simulink model "GCU_Model_genCode"  (R2018a)
settings: Solver=FixedStepDiscrete  StartTime=0.0  StopTime=20  FixedStep=0.0001  RelTol=1e-3  EnableMultiTasking=on
undefined symbols (not defined in the file): ConversionGainVector, ConversionOffsetVector, VoltageGainVector, VoltageOffsetVector
libraries: canLib x5, simulink x5, uartLib x2, utilityLib x1, clutchMotorLib x1, efiLib x1, engineControlLib x1, cstblocks x1, gearMotorLib x1
(part 2 of 3)

== system GCU_Model_genCode/EEPROM/Evaluate_Request/Read ==
  page : Inport
  cell : Inport  Port=2
  dataSize : Inport  Port=3
  Action Port : ActionPort  ActionType=elseif
  Eeprom_read : S-Function  FunctionName=Eeprom_read  SFunctionDeploymentMode=off  EnableBusSupport=off
  readResult : Outport
  data : Outport  Port=2
  wires:
  Eeprom_read/1 -> readResult/1
  Eeprom_read/2 -> data/1
  page/1 -> Eeprom_read/1
  cell/1 -> Eeprom_read/2
  dataSize/1 -> Eeprom_read/3

== system GCU_Model_genCode/EEPROM/Evaluate_Request/Write ==
  page : Inport
  cell : Inport  Port=2
  dataSize : Inport  Port=3
  data : Inport  Port=4
  Action Port : ActionPort  ActionType=then
  Eeprom_write : S-Function  FunctionName=Eeprom_write  SFunctionDeploymentMode=off  EnableBusSupport=off
  writeResult : Outport
  wpState : Outport  Port=2
  wires:
  cell/1 -> Eeprom_write/2
  page/1 -> Eeprom_write/1
  dataSize/1 -> Eeprom_write/3
  data/1 -> Eeprom_write/4
  Eeprom_write/2 -> wpState/1
  Eeprom_write/1 -> writeResult/1

== system GCU_Model_genCode/GCU_CAN_Read/MessageEvaluation1/setMap/If Action Subsystem ==
  In1 : Inport
  Action Port : ActionPort  ActionType=then
  Out1 : Outport
  wires:
  In1/1 -> Out1/1

== system GCU_Model_genCode/GCU_CAN_Read/MessageEvaluation1/setMap/If Action Subsystem1 ==
  In1 : Inport
  Action Port : ActionPort  ActionType=else
  Out1 : Outport
  wires:
  In1/1 -> Out1/1

== system GCU_Model_genCode/GCU_timer/Anti_Stall_System/antiStallLogic/AntiStallActivate ==
  Inport : Inport
  f : TriggerPort  TriggerType=function-call  VariantControl=(inherit)
      settings: CopyFcn=Stateflow.SLINSF.SimulinkMan.removeBlockPreDeleteFcn  PreDeleteFcn=Stateflow.SLINSF.SimulinkMan.unsafePredeleteFcn
  ClutchMotor SetPosition : S-Function  FunctionName=ClutchMotor_setPosition  SFunctionDeploymentMode=off  EnableBusSupport=off
  wires:
  Inport/1 -> ClutchMotor SetPosition/1

== stateflow chart GCU_Model_genCode/GCU_timer/GCULogic ==
  settings: updateMethod=DISCRETE  sampleTime=0.001
  state MODES [parallel]
    settings: executionOrder=1
    state MANUAL_MODES
      entry:
      lastModeCom[0] = modeCom[0];
      lastModeCom[1] = modeCom[1];
      entry, during:
      checkShift();
      checkClutch();
      state ENDURANCE
      state SKIDPAD
      (default) -> ENDURANCE
    state INIT
      entry:
      send(BuzzerOn);
      during:
      buzzerCounter++;
    note: azzerare nel modo giusto i feedback e i comandi
    note: POSSIAMO FARLO UGUALE PER ACCELERATION E AUTOX?
    state checkClutch [function]
      (default) -> (junction 649)
      (junction 649) -> (junction 648) [order 1] : [clutchTarget ~= clutchCurrVal && antiStallFb == ANTISTALL_OFF]
      (junction 649) -> (junction 683) [order 2]
      (junction 648) -> (junction 682)
      (junction 682) -> (junction 687) [order 1] : [(~in(GEARSHIFT.DOWNSHIFTING) && ~in(NEUTRAL_STATE.SET_NEUTRAL)) || in(NEUTRAL_STATE.UNSET_NEUTRAL)]
      (junction 682) -> (junction 689) [order 2]
      (junction 687) -> (junction 691) : {Clutch_setValue(clutchTarget);}
    note: In caso di problema si riporta in endurance
    state checkShift [function]
      (default) -> (junction 635)
      (junction 635) -> (junction 637) [order 1] : [shiftCom[0] ~= lastShiftCom]
      (junction 635) -> (junction 641) [order 2]
      (junction 637) -> (junction 448) : {lastShiftCom = shiftCom[0];}
      (junction 448) -> (junction 450) [order 1] : [ shiftCom[1] == GEAR_COMMAND_UP]
      (junction 448) -> (junction 454) [order 2]
      (junction 450) -> (junction 452) : {send(GearshiftUp, NEUTRAL_STATE);
          |  send(GearshiftUp, GEARSHIFT);}
      (junction 454) -> (junction 456) [order 1] : [shiftCom[1] == GEAR_COMMAND_DOWN]
      (junction 454) -> (junction 460) [order 2]
      (junction 456) -> (junction 458) : {send(GearshiftDown, NEUTRAL_STATE);
          |  send(GearshiftDown, GEARSHIFT);}
      (junction 460) -> (junction 462) [order 1] : [shiftCom[1] == GEAR_COMMAND_NEUTRAL_UP]
      (junction 460) -> (junction 466) [order 2]
      (junction 462) -> (junction 464) : {send(GearshiftSetNeutral, NEUTRAL_STATE);
          |  send(GearshiftUp, GEARSHIFT);}
      (junction 466) -> (junction 469) [order 1] : [shiftCom[1] == GEAR_COMMAND_NEUTRAL_DOWN]
      (junction 466) -> (junction 473) [order 2]
      (junction 469) -> (junction 471) : {send(GearshiftSetNeutral, NEUTRAL_STATE);
          |  send(GearshiftDown, GEARSHIFT); }
    state ACCELERATION
      entry:
      lastAacCom = aacCom[0];
      lastModeCom[0] = modeCom[0];
      lastModeCom[1] = modeCom[1];
      note: ClutchSet si annulla se provo a tirarla in ready?
      state ACC
        note: Ricorda load dei default parameters
        note: Forse serve stato OFF, forse no
        note: ATTENZIONE: mancano delle istruzioni in alcuni stati
        note: E' giusto che clutch venga settata due volte?
        note: Riguarda funzionamento counter
        state ACTIVE
          note: Quindi continuo a settare Clutch?
          state START
            entry:
            stateFb = ACC_READY;
            aacCounter = AAC_WORK_RATE_ms
            send(Efi_setRPMLimiter);
            Clutch_setValue(uint8(100));
            during:
            aacCounter = aacCounter - 1;
          state READY
            entry:
            stateFb = ACC_READY;
            aacCounter = AAC_WORK_RATE_ms
            Clutch_setValue(uint8(100));
            during:
            aacCounter = aacCounter - 1;
            en, du:
            checkShift();
          note: SET blip è sbagliato
          state START_RELEASE
            entry:
            stateFb = ACC_GO;
            aac_clutchValue = double(getAacParam(acc_params.RAMP_START));
            Clutch_setValue(uint8(aac_clutchValue));
            aac_dtRelease = getAacParam(acc_params.RAMP_TIME) / int32(AAC_WORK_RATE_ms);
            aac_clutchStep = double((getAacParam(acc_params.RAMP_START) - getAacParam(acc_params.RAMP_END)) * int32(AAC_WORK_RATE_ms)) / double(getAacParam(acc_params.RAMP_TIME));
            aacCounter = AAC_WORK_RATE_ms;
            during:
            aacCounter = aacCounter - 1;
          state RUNNING
            entry:
            aacCounter = AAC_WORK_RATE_ms
            lastShift =  currentGear;
            entry, during:
            aacCheckShift();
          note: Continuo a controllare ogni 25ms?
          state aacCheckShift [function]
            (default) -> (junction 716)
            (junction 716) -> (junction 717) [order 1] : [lastShift == currentGear]
            (junction 716) -> (junction 720) [order 2]
            (junction 717) -> (junction 593)
            (junction 593) -> (junction 604) [order 1] : [acc_externValues[int32(acc_values.RPM)] >= acc_parameters[ uint8(acc_params.RPM_LIMIT_1_2) + currentGear -1]]
            (junction 593) -> (junction 606) [order 2]
            (junction 604) -> (junction 608)
            (junction 608) -> (junction 610) [order 1] : [acc_externValues[int32(acc_values.WHEEL_SPEED)] >= acc_parameters[ uint8(acc_params.SPEED_LIMIT_1_2) + currentGear-1]]
            (junction 608) -> (junction 612) [order 2]
            (junction 610) -> (junction 614) : {send(GearshiftUp, GEARSHIFT); lastShift = lastShift + 1;}
          state RELEASING
            entry:
            aac_clutchValue = aac_clutchValue - aac_clutchStep;
            Clutch_setValue(uint8(aac_clutchValue));
            aac_dtRelease = aac_dtRelease - 1;
            aacCounter = AAC_WORK_RATE_ms;
            during:
            aacCounter = aacCounter - 1;
          note: Teniamo questa cosa di eseguire ogni 25ms? O calcoliamo direttamente
              | il Ttot?
          (default) -> MODES.ACCELERATION.ACC.ACTIVE.START
          (junction 558) -> MODES.ACCELERATION.ACC.ACTIVE.READY [order 2]
          MODES.ACCELERATION.ACC.ACTIVE.START -> MODES.ACCELERATION.ACC.ACTIVE.READY : [aacCounter <= 1]
          MODES.ACCELERATION.ACC.ACTIVE.READY -> (junction 558) : [aacCounter <= 1]
          (junction 558) -> MODES.ACCELERATION.ACC.ACTIVE.START_RELEASE [order 1] : [aacCom[0] ~= lastAacCom && aacCom[1] == ACC_GO && acc_externValues[int32(acc_values.TPS)] >= getAacParam(acc_params.TPS_START_LIMIT) ]{lastAacCom = aacCom[0];}
          MODES.ACCELERATION.ACC.ACTIVE.START_RELEASE -> MODES.ACCELERATION.ACC.ACTIVE.RELEASING : [aacCounter <= 1]
          (junction 572) -> MODES.ACCELERATION.ACC.ACTIVE.RUNNING [order 1] : [aac_dtRelease <= 0 || clutchCurrVal <= getAacParam(acc_params.RAMP_END)]
              | {Clutch_setValue(uint8(0)); send(Efi_unsetRPMLimiter);}
          (junction 572) -> MODES.ACCELERATION.ACC.ACTIVE.RELEASING [order 2]
          MODES.ACCELERATION.ACC.ACTIVE.RELEASING -> (junction 572) : [aacCounter <=1]
        note: Quando devo fare clutch release?Forse risolto in CAN
        state STOPPING
          entry:
          send(Efi_unsetRPMLimiter);
          Clutch_setValue(uint8(0));
          //sendUpdatesSW(ACC_CODE, uint16(0));
        note: da verificare la marcia di uscita
        note: !!!!Gli array di MATLAB sono 1-based
        state param = getAacParam(index) [function]
          (default) -> (junction 566)
          (junction 566) -> (junction 570) : {param = acc_parameters[int32(index)]}
        MODES.ACCELERATION.ACC.ACTIVE -> MODES.ACCELERATION.ACC.STOPPING : [aacCom[0] ~= lastAacCom && aacCom[1] == ACC_OFF]
            | {lastAacCom = aacCom[0]}
        MODES.ACCELERATION.ACC.ACTIVE.RUNNING -> MODES.ACCELERATION.ACC.STOPPING : [currentGear >= 5 && currentGear != 8]
      state DEFAULT
        entry, during:
        stateFb = ACC_OFF;
        checkShift();
        checkClutch();
      note: prima di entrare svuotare il buffer
      (default) -> MODES.ACCELERATION.DEFAULT
      MODES.ACCELERATION.DEFAULT -> MODES.ACCELERATION.ACC.ACTIVE : [aacCom[0] ~= lastAacCom && aacCom[1] == ACC_READY]
          | {lastAacCom = aacCom[0]}
      MODES.ACCELERATION.ACC.STOPPING -> MODES.ACCELERATION.DEFAULT
    note: il controllo se fare stopAcc in caso di comando di cambio meglio farlo dentro aac e non in CAN evaluation
    state AUTOCROSS
      entry:
      lastAutoXCom = autoXCom[0];
      lastModeCom[0] = modeCom[0];
      lastModeCom[1] = modeCom[1];
      state LAUNCH
        note: Ricorda load dei default parameters
        note: Forse serve stato OFF, forse no
        state ACTIVE
          note: TOGLIAMO STA COSA DEL WORK RATE?
          state START
            entry:
            stateFb = AUTOX_READY;
            autoXCounter = AUTOX_WORK_RATE_ms
            send(Efi_setRPMLimiter);
            Clutch_setValue(uint8(100));
            during:
            autoXCounter = autoXCounter - 1;
          state READY
            entry:
            stateFb = AUTOX_READY;
            autoXCounter = AUTOX_WORK_RATE_ms
            Clutch_setValue(uint8(100));
            during:
            autoXCounter = autoXCounter - 1;
            en, du:
            checkShift();
          state START_RELEASE
            entry:
            stateFb = AUTOX_GO;
            autoX_clutchValue = double(getAutoXParam(AUTOX_RAMP_START));
            Clutch_setValue(uint8(autoX_clutchValue));
            autoX_dtRelease = getAutoXParam(AUTOX_RAMP_TIME) / int32(AUTOX_WORK_RATE_ms);
            autoX_clutchStep = double((getAutoXParam(AUTOX_RAMP_START) - getAutoXParam(AUTOX_RAMP_END)) * int32(AUTOX_WORK_RATE_ms)) / double(getAutoXParam(AUTOX_RAMP_TIME));
            autoXCounter = AUTOX_WORK_RATE_ms;
            during:
            autoXCounter = autoXCounter - 1;
          state RUNNING
            entry:
            autoXCounter = AUTOX_WORK_RATE_ms
            lastShift =  currentGear;
            entry, during:
            autoXCheckShift();
          state autoXCheckShift [function]
            (default) -> (junction 1005)
            (junction 1005) -> (junction 1006) [order 1] : [lastShift == currentGear]
            (junction 1005) -> (junction 1007) [order 2]
            (junction 1006) -> (junction 1008)
            (junction 1008) -> (junction 1009) [order 1] : [acc_externValues[int32(acc_values.RPM)] >= autoX_parameters[ uint8(AUTOX_RPM_LIMIT_1_2) + currentGear -1]]
            (junction 1008) -> (junction 1010) [order 2]
            (junction 1009) -> (junction 1011)
            (junction 1011) -> (junction 1012) [order 1] : [acc_externValues[int32(acc_values.WHEEL_SPEED)] >= autoX_parameters[ uint8(AUTOX_SPEED_LIMIT_1_2) + currentGear-1]]
            (junction 1011) -> (junction 1014) [order 2]
            (junction 1012) -> (junction 1013) : {send(GearshiftUp, GEARSHIFT); lastShift = lastShift + 1;}
          state RELEASING
            entry:
            autoX_clutchValue = autoX_clutchValue - autoX_clutchStep;
            Clutch_setValue(uint8(autoX_clutchValue));
            autoX_dtRelease = autoX_dtRelease - 1;
            autoXCounter = AUTOX_WORK_RATE_ms;
            during:
            autoXCounter = autoXCounter - 1;
          (default) -> MODES.AUTOCROSS.LAUNCH.ACTIVE.START
          (junction 986) -> MODES.AUTOCROSS.LAUNCH.ACTIVE.READY [order 2]
          MODES.AUTOCROSS.LAUNCH.ACTIVE.START -> MODES.AUTOCROSS.LAUNCH.ACTIVE.READY : [autoXCounter <= 1]
          MODES.AUTOCROSS.LAUNCH.ACTIVE.READY -> (junction 986) : [autoXCounter <= 1]
          (junction 986) -> MODES.AUTOCROSS.LAUNCH.ACTIVE.START_RELEASE [order 1] : [autoXCom[0] ~= lastAutoXCom && autoXCom[1] == AUTOX_GO && acc_externValues[int32(acc_values.TPS)] >= getAutoXParam(AUTOX_TPS_START_LIMIT) ]{lastAutoXCom = autoXCom[0];}
          MODES.AUTOCROSS.LAUNCH.ACTIVE.START_RELEASE -> MODES.AUTOCROSS.LAUNCH.ACTIVE.RELEASING : [autoXCounter <= 1]
          (junction 987) -> MODES.AUTOCROSS.LAUNCH.ACTIVE.RUNNING [order 1] : [autoX_dtRelease <= 0 || clutchCurrVal <= getAutoXParam(AUTOX_RAMP_END)]
              | {Clutch_setValue(uint8(0)); send(Efi_unsetRPMLimiter);}
          (junction 987) -> MODES.AUTOCROSS.LAUNCH.ACTIVE.RELEASING [order 2]
          MODES.AUTOCROSS.LAUNCH.ACTIVE.RELEASING -> (junction 987) : [autoXCounter <=1]
        note: Quando devo fare clutch release?Forse risolto in CAN
        state STOPPING
          entry:
          send(Efi_unsetRPMLimiter);
          Clutch_setValue(uint8(0));
        note: da verificare la marcia di uscita
        note: !!!!Gli array di MATLAB sono 1-based
        state param = getAutoXParam(index) [function]
          (default) -> (junction 1034)
          (junction 1034) -> (junction 1035) : {param = autoX_parameters[int32(index)]}
        MODES.AUTOCROSS.LAUNCH.ACTIVE -> MODES.AUTOCROSS.LAUNCH.STOPPING : [autoXCom[0] ~= lastAutoXCom && autoXCom[1] == AUTOX_DEFAULT]
            | {lastAutoXCom = autoXCom[0]}
        MODES.AUTOCROSS.LAUNCH.ACTIVE.RUNNING -> MODES.AUTOCROSS.LAUNCH.STOPPING : [currentGear >= 3 && currentGear != 8]
      state DEFAULT
        entry, during:
        stateFb = AUTOX_DEFAULT;
        checkShift();
        checkClutch();
      note: TOGLIAMO STA COSA DEL WORK RATE?
      (default) -> MODES.AUTOCROSS.DEFAULT
      MODES.AUTOCROSS.DEFAULT -> MODES.AUTOCROSS.LAUNCH.ACTIVE : [autoXCom[0] ~= lastAutoXCom && autoXCom[1] == AUTOX_READY]
          | {lastAutoXCom = autoXCom[0]}
      MODES.AUTOCROSS.LAUNCH.STOPPING -> MODES.AUTOCROSS.DEFAULT
    state ACCELERATION_PID
      entry:
      lastAutoXCom = autoXCom[0];
      lastModeCom[0] = modeCom[0];
      lastModeCom[1] = modeCom[1];
      state LAUNCH
        note: Ricorda load dei default parameters
        note: Forse serve stato OFF, forse no
        state ACTIVE
          note: TOGLIAMO STA COSA DEL WORK RATE?
          state START
            entry:
            stateFb = AUTOX_READY;
            autoXCounter = AUTOX_WORK_RATE_ms
            send(Efi_setRPMLimiter);
            Clutch_setValue(uint8(100));
            during:
            autoXCounter = autoXCounter - 1;
          state READY
            entry:
            stateFb = AUTOX_READY;
            autoXCounter = AUTOX_WORK_RATE_ms
            Clutch_setValue(uint8(55));
            during:
            autoXCounter = autoXCounter - 1;
            en, du:
            checkShift();
          state RUNNING
            entry:
            autoXCounter = AUTOX_WORK_RATE_ms
            lastShift =  currentGear;
            entry, during:
            autoXCheckShift();
          state RELEASE
            entry:
            pidControl(SLIP_TARGET, currSlip,1);
            state Control
              entry:
              clutchCurrVal = pidControl(SLIP_TARGET, currSlip[1], 0);
            state WAIT
            (default) -> MODES.ACCELERATION_PID.LAUNCH.ACTIVE.RELEASE.WAIT
            MODES.ACCELERATION_PID.LAUNCH.ACTIVE.RELEASE.WAIT -> Control : [currSlip[0] != lastSlip]{lastSlip = currSlip[0];}
            Control -> MODES.ACCELERATION_PID.LAUNCH.ACTIVE.RELEASE.WAIT
          state autoXCheckShift [function]
            (default) -> (junction 1124)
            (junction 1124) -> (junction 1125) [order 1] : [lastShift == currentGear]
            (junction 1124) -> (junction 1126) [order 2]
            (junction 1125) -> (junction 1127)
            (junction 1127) -> (junction 1128) [order 1] : [acc_externValues[int32(acc_values.RPM)] >= autoX_parameters[ uint8(AUTOX_RPM_LIMIT_1_2) + currentGear -1]]
            (junction 1127) -> (junction 1129) [order 2]
            (junction 1128) -> (junction 1130)
            (junction 1130) -> (junction 1131) [order 1] : [acc_externValues[int32(acc_values.WHEEL_SPEED)] >= autoX_parameters[ uint8(AUTOX_SPEED_LIMIT_1_2) + currentGear-1]]
            (junction 1130) -> (junction 1133) [order 2]
            (junction 1131) -> (junction 1132) : {send(GearshiftUp, GEARSHIFT); lastShift = lastShift + 1;}
          state clutchVal = pidControl(slipTarget,currentSlip,reset) [function]
          (default) -> MODES.ACCELERATION_PID.LAUNCH.ACTIVE.START
          (junction 1107) -> MODES.ACCELERATION_PID.LAUNCH.ACTIVE.READY [order 2]
          MODES.ACCELERATION_PID.LAUNCH.ACTIVE.START -> MODES.ACCELERATION_PID.LAUNCH.ACTIVE.READY : [autoXCounter <= 1]
          MODES.ACCELERATION_PID.LAUNCH.ACTIVE.READY -> (junction 1107) : [autoXCounter <= 1]
          (junction 1107) -> RELEASE [order 1] : [autoXCom[0] ~= lastAutoXCom && autoXCom[1] == AUTOX_GO && acc_externValues[int32(acc_values.TPS)] >= getAutoXParam(AUTOX_TPS_START_LIMIT) ]{lastAutoXCom = autoXCom[0]; stateFb = AUTOX_GO;}
          RELEASE -> MODES.ACCELERATION_PID.LAUNCH.ACTIVE.RUNNING : [acc_externValues[int32(acc_values.WHEEL_SPEED)] >= RELEASE_END_SPEED]{Clutch_setValue(uint8(0)); send(Efi_unsetRPMLimiter);}
        note: Quando devo fare clutch release?Forse risolto in CAN
        state STOPPING
          entry:
          send(Efi_unsetRPMLimiter);
          Clutch_setValue(uint8(0));
        note: da verificare la marcia di uscita
        note: !!!!Gli array di MATLAB sono 1-based
        state param = getAutoXParam(index) [function]
          (default) -> (junction 1152)
          (junction 1152) -> (junction 1153) : {param = autoX_parameters[int32(index)]}
        MODES.ACCELERATION_PID.LAUNCH.ACTIVE -> MODES.ACCELERATION_PID.LAUNCH.STOPPING : [autoXCom[0] ~= lastAutoXCom && autoXCom[1] == AUTOX_DEFAULT]
            | {lastAutoXCom = autoXCom[0]}
        MODES.ACCELERATION_PID.LAUNCH.ACTIVE.RUNNING -> MODES.ACCELERATION_PID.LAUNCH.STOPPING : [currentGear >= 3 && currentGear != 8]
      state DEFAULT
        entry, during:
        stateFb = AUTOX_DEFAULT;
        checkShift();
        checkClutch();
      (default) -> MODES.ACCELERATION_PID.DEFAULT
      MODES.ACCELERATION_PID.DEFAULT -> MODES.ACCELERATION_PID.LAUNCH.ACTIVE : [autoXCom[0] ~= lastAutoXCom && autoXCom[1] == AUTOX_READY]
          | {lastAutoXCom = autoXCom[0]}
      MODES.ACCELERATION_PID.LAUNCH.STOPPING -> MODES.ACCELERATION_PID.DEFAULT
    (junction 826) -> (junction 808)
    (default) -> MODES.INIT
    MODES.INIT -> (junction 808) : [buzzerCounter>=1000]{send(BuzzerOff);}
    (junction 808) -> ENDURANCE [order 1] : [modeCom[1] == ENDURANCE_MODE]
    (junction 808) -> (junction 812) [order 2]
    MANUAL_MODES -> (junction 826) : [modeCom[0] != lastModeCom[0] && modeCom[1] != lastModeCom[1]]
    AUTOCROSS -> (junction 826) : [modeCom[0]~= lastModeCom[0] && modeCom[1] != lastModeCom[1]]
        | {send(Efi_unsetRPMLimiter);
        |   stateFb = ACC_OFF;
        |   Clutch_setValue(uint8(0));}
    ACCELERATION -> (junction 826) : [modeCom[0]~= lastModeCom[0] && modeCom[1] != lastModeCom[1]]
        | {send(Efi_unsetRPMLimiter);
        |   stateFb = ACC_OFF;
        |   Clutch_setValue(uint8(0));}
    (junction 812) -> SKIDPAD [order 1] : [modeCom[1] == SKIDPAD_MODE]
    (junction 812) -> (junction 815) [order 2]
    (junction 1159) -> MANUAL_MODES [order 2]
    (junction 815) -> ACCELERATION [order 1] : [modeCom[1] == ACCELERATION_MODE]
    (junction 815) -> (junction 1039) [order 2]
    (junction 1039) -> AUTOCROSS [commented out] : [modeCom[1] == AUTOX_MODE]
    (junction 1039) -> (junction 1159)
    (junction 1159) -> ACCELERATION_PID [order 1] : [modeCom[1] == AUTOX_MODE]
  state NEUTRAL_STATE [parallel]
    settings: executionOrder=2
    state NEUTRAL
    state UNSET_NEUTRAL
    state SET_NEUTRAL
    state NO_NEUTRAL
    NEUTRAL -> UNSET_NEUTRAL [order 2] : GearshiftDown
    (default) -> NEUTRAL
    NEUTRAL -> UNSET_NEUTRAL [order 1] : GearshiftUp
    SET_NEUTRAL -> NEUTRAL : [in(GEARSHIFT.DOWN_END) || in(GEARSHIFT.UP_END)]
    NEUTRAL -> NO_NEUTRAL [order 3] : [currentGear != 0]
    UNSET_NEUTRAL -> NO_NEUTRAL : [in(GEARSHIFT.DOWN_END) || in(GEARSHIFT.UP_END)]
    NO_NEUTRAL -> SET_NEUTRAL : GearshiftSetNeutral
  state GEARSHIFT [parallel]
    settings: executionOrder=3
    state UPSHIFTING
      state UP_REBOUND
        entry:
        ticksCounter = Gearshift_getTime();
        during:
        ticksCounter = ticksCounter - 1;
        state Default
          entry:
          send(Gearshift_rebound);
        state SettingNeutral
          entry:
          Clutch_setValue(uint8(0));
          send(Gearshift_rebound);
        (default) -> (junction 392)
        (junction 392) -> GEARSHIFT.UPSHIFTING.UP_REBOUND.Default [order 2]
        (junction 392) -> GEARSHIFT.UPSHIFTING.UP_REBOUND.SettingNeutral [order 1] : [in(NEUTRAL_STATE.SET_NEUTRAL)]
      state UP_PUSH
        entry:
        ticksCounter = Gearshift_getTime();
        during:
        ticksCounter = ticksCounter - 1;
        state Default
          entry:
          send(Gearshift_up_push);
        state CutOff
          entry:
          send(Efi_unsetCut);
          send(Gearshift_up_push);
        (default) -> (junction 424)
        (junction 424) -> GEARSHIFT.UPSHIFTING.UP_PUSH.Default [order 2]
        (junction 424) -> CutOff [order 1] : [~in(NEUTRAL_STATE.SET_NEUTRAL)]
      state UP_START
        entry:
        ticksCounter = Gearshift_getTime() + 1;
        during:
        ticksCounter = ticksCounter - 1;
        state Default
          entry:
          Efi_setCut;
        state SettingNeutral
          entry:
          Clutch_setValue(uint8(80));
        (default) -> (junction 386)
        (junction 386) -> GEARSHIFT.UPSHIFTING.UP_START.Default [order 2]
        (junction 386) -> GEARSHIFT.UPSHIFTING.UP_START.SettingNeutral [order 1] : [in(NEUTRAL_STATE.SET_NEUTRAL)]
      state UP_BRAKE
        entry:
        ticksCounter = Gearshift_getTime();
        send(Gearshift_brake);
        during:
        ticksCounter = ticksCounter - 1;
      UP_REBOUND -> UP_BRAKE : [ticksCounter == 1]
      UP_START -> UP_PUSH : [ticksCounter == 1]
      UP_PUSH -> UP_REBOUND : [ticksCounter == 1]
    note: +1 da aggiungere solo qui per correggere come gli stati entry vengono eseguiti in c (in contemporanea alla exit dello stato precedente
    state UP_END
      entry:
      send(Gearshift_free);
    state IDLE
    state INIT
      entry:
      ticksCounter = 0;
    note: Ricorda inizializzare CLUTCH
    state DOWNSHIFTING
      state DOWN_START
        entry:
        ticksCounter = Gearshift_getTime();
        during:
        ticksCounter = ticksCounter - 1;
        state SettingNeutral
          entry:
          Clutch_setValue(uint8(80));
        state ChangeClutch
          entry:
          Clutch_setValue(uint8(60));
        state Default
        (default) -> (junction 400)
        (junction 400) -> GEARSHIFT.DOWNSHIFTING.DOWN_START.SettingNeutral [order 1] : [in(NEUTRAL_STATE.SET_NEUTRAL)  &&  clutchCurrVal <= 80]
        (junction 400) -> (junction 403) [order 2]
        (junction 403) -> GEARSHIFT.DOWNSHIFTING.DOWN_START.ChangeClutch [order 1] : [~in(NEUTRAL_STATE.UNSET_NEUTRAL) && clutchCurrVal <= 60]
        (junction 403) -> GEARSHIFT.DOWNSHIFTING.DOWN_START.Default [order 2]
      state DOWN_BRAKE
        entry:
        ticksCounter =Gearshift_getTime();
        during:
        ticksCounter = ticksCounter - 1;
        state Default
          entry:
          send(Gearshift_brake);
        state ChangeClutch
          entry:
          Clutch_setValue(uint8(80));
          send(Gearshift_brake);
        (default) -> (junction 411)
        (junction 411) -> GEARSHIFT.DOWNSHIFTING.DOWN_BRAKE.Default [order 2]
        (junction 411) -> GEARSHIFT.DOWNSHIFTING.DOWN_BRAKE.ChangeClutch [order 1] : [clutchCurrVal < 81]
      state DOWN_PUSH
        entry:
        ticksCounter = Gearshift_getTime();
        send(Gearshift_down_push);
        during:
        ticksCounter = ticksCounter - 1;
      state DOWN_REBOUND
        entry:
        ticksCounter = Gearshift_getTime();
        send(Gearshift_rebound);
        during:
        ticksCounter = ticksCounter - 1;
      DOWN_START -> DOWN_PUSH : [ticksCounter == 1]
      DOWN_REBOUND -> DOWN_BRAKE : [ticksCounter == 1]
      DOWN_PUSH -> DOWN_REBOUND : [ticksCounter == 1]
    state DOWN_END
      entry:
      send(Gearshift_free);
    state time = Gearshift_getTime [function]
      (default) -> (junction 238)
      (junction 238) -> (junction 240) [order 1] : [in(UPSHIFTING.UP_START)]
      (junction 240) -> (junction 271) [order 1] : [in(NEUTRAL_STATE.SET_NEUTRAL)]
      (junction 240) -> (junction 322) [order 2] : {time = int32(timings[DELAY]);}
      (junction 271) -> (junction 275) : {time = int32(timings[DEFAULT_NT_CLUTCH_DELAY]);}
      (junction 238) -> (junction 241) [order 2]
      (junction 241) -> (junction 347) [order 1] : [in(UPSHIFTING.UP_PUSH)]
      (junction 347) -> (junction 348) [order 1] : [in(NEUTRAL_STATE.SET_NEUTRAL)]
      (junction 347) -> (junction 359) [order 2]
      (junction 348) -> (junction 363) : {time = int32(timings[NT_CLUTCH_DELAY])}
      (junction 241) -> (junction 243) [order 2]
      (junction 243) -> (junction 244) [order 1] : [in(UPSHIFTING.UP_REBOUND)]
      (junction 244) -> (junction 324) [order 1] : [in(NEUTRAL_STATE.SET_NEUTRAL)]
      (junction 243) -> (junction 245) [order 2]
      (junction 244) -> (junction 326) [order 2] : {time = int32(timings[UP_REBOUND]);}
      (junction 324) -> (junction 327) : {time = int32(timings[NT_REBOUND_1_N]);}
      (junction 359) -> (junction 360) [order 1] : [currentGear == 1]
      (junction 360) -> (junction 365) : {time = int32(timings[UP_PUSH_1_2])}
      (junction 359) -> (junction 351) [order 2]
      (junction 245) -> (junction 246) [order 1] : [in(UPSHIFTING.UP_BRAKE)]
      (junction 246) -> (junction 330) [order 1] : [in(NEUTRAL_STATE.SET_NEUTRAL)]
      (junction 351) -> (junction 362) [order 1] : [currentGear == 2]
      (junction 362) -> (junction 367) : {time = int32(timings[UP_PUSH_2_3])}
      (junction 245) -> (junction 247) [order 2]
      (junction 246) -> (junction 332) [order 2] : {time = int32(timings[UP_BRAKE]);}
      (junction 330) -> (junction 333) : {time = int32(timings[NT_BRAKE_1_N]);}
      (junction 351) -> (junction 355) [order 2]
      (junction 247) -> (junction 248) [order 1] : [in(DOWNSHIFTING.DOWN_START)]
      (junction 355) -> (junction 344) [order 1] : [currentGear == 3]
      (junction 344) -> (junction 369) : {time = int32(timings[UP_PUSH_3_4])}
      (junction 247) -> (junction 249) [order 2]
      (junction 248) -> (junction 336) : {time = int32(timings[CLUTCH]);}
      (junction 355) -> (junction 356) [order 2]
      (junction 249) -> (junction 250) [order 1] : [in(DOWNSHIFTING.DOWN_PUSH)]
      (junction 356) -> (junction 354) [order 1] : [currentGear == 4]
      (junction 354) -> (junction 371) : {time = int32(timings[UP_PUSH_4_5])}
      (junction 249) -> (junction 251) [order 2]
      (junction 250) -> (junction 338) : {time = int32(timings[DN_PUSH]);}
      (junction 356) -> (junction 342) [order 2] : {time = int32(timings[UP_PUSH_2_3])}
      (junction 251) -> (junction 252) [order 1] : [in(DOWNSHIFTING.DOWN_REBOUND)]
      (junction 251) -> (junction 254) [order 2] : {time = int32(timings[DN_BRAKE]);}
      (junction 252) -> (junction 340) : {time = int32(timings[DN_REBOUND]);}
    state time = Gearshift_getTime_old [function] [commented out]
      (default) -> (junction 841) [commented out]
      (junction 841) -> (junction 842) [commented out] : [in(UPSHIFTING.UP_START)]
      (junction 842) -> (junction 843) [commented out] : [in(NEUTRAL_STATE.SET_NEUTRAL)]
      (junction 841) -> (junction 846) [commented out]
      (junction 842) -> (junction 844) [commented out] : {time = int32(timings.DEFAULT_DELAY);}
      (junction 843) -> (junction 845) [commented out] : {time = int32(timings.DEFAULT_NT_CLUTCH_DELAY);}
      (junction 846) -> (junction 847) [commented out] : [in(UPSHIFTING.UP_PUSH)]
      (junction 847) -> (junction 848) [commented out] : [in(NEUTRAL_STATE.SET_NEUTRAL)]
      (junction 847) -> (junction 853) [commented out]
      (junction 848) -> (junction 852) [commented out] : {time = int32(timings.DEFAULT_NT_CLUTCH_DELAY)}
      (junction 846) -> (junction 850) [commented out]
      (junction 850) -> (junction 851) [commented out] : [in(UPSHIFTING.UP_REBOUND)]
      (junction 851) -> (junction 849) [commented out] : [in(NEUTRAL_STATE.SET_NEUTRAL)]
      (junction 850) -> (junction 859) [commented out]
      (junction 851) -> (junction 855) [commented out] : {time = int32(timings.DEFAULT_UP_REBOUND);}
      (junction 849) -> (junction 856) [commented out] : {time = int32(timings.DEFAULT_NT_REBOUND_1_N);}
      (junction 853) -> (junction 854) [commented out] : [currentGear == 1]
      (junction 854) -> (junction 857) [commented out] : {time = int32(timings.DEFAULT_UP_PUSH_1_2)}
      (junction 853) -> (junction 858) [commented out]
      (junction 859) -> (junction 860) [commented out] : [in(UPSHIFTING.UP_BRAKE)]
      (junction 860) -> (junction 861) [commented out] : [in(NEUTRAL_STATE.SET_NEUTRAL)]
      (junction 858) -> (junction 862) [commented out] : [currentGear == 2]
      (junction 862) -> (junction 865) [commented out] : {time = int32(timings.DEFAULT_UP_PUSH_2_3)}
      (junction 859) -> (junction 867) [commented out]
      (junction 860) -> (junction 863) [commented out] : {time = int32(timings.DEFAULT_UP_BRAKE);}
      (junction 861) -> (junction 864) [commented out] : {time = int32(timings.DEFAULT_NT_BRAKE_1_N);}
      (junction 858) -> (junction 866) [commented out]
      (junction 867) -> (junction 868) [commented out] : [in(DOWNSHIFTING.DOWN_START)]
      (junction 866) -> (junction 869) [commented out] : [currentGear == 3]
      (junction 869) -> (junction 871) [commented out] : {time = int32(timings.DEFAULT_UP_PUSH_3_4)}
      (junction 867) -> (junction 873) [commented out]
      (junction 868) -> (junction 870) [commented out] : {time = int32(timings.DEFAULT_CLUTCH);}
      (junction 866) -> (junction 872) [commented out]
      (junction 873) -> (junction 874) [commented out] : [in(DOWNSHIFTING.DOWN_PUSH)]
      (junction 872) -> (junction 875) [commented out] : [currentGear == 4]
      (junction 875) -> (junction 877) [commented out] : {time = int32(timings.DEFAULT_UP_PUSH_4_5)}
      (junction 873) -> (junction 878) [commented out]
      (junction 874) -> (junction 876) [commented out] : {time = int32(timings.DEFAULT_DN_PUSH);}
      (junction 872) -> (junction 881) [commented out] : {time = int32(timings.DEFAULT_UP_PUSH_2_3)}
      (junction 878) -> (junction 879) [commented out] : [in(DOWNSHIFTING.DOWN_REBOUND)]
      (junction 878) -> (junction 882) [commented out] : {time = int32(timings.DEFAULT_DN_BRAKE);}
      (junction 879) -> (junction 880) [commented out] : {time = int32(timings.DEFAULT_DN_REBOUND);}
    IDLE -> UP_START [order 1] : GearshiftUp[currentGear < 5]
    UP_BRAKE -> UP_END : [ticksCounter == 1]
    UP_END -> IDLE
    (default) -> GEARSHIFT.INIT
    GEARSHIFT.INIT -> IDLE
    DOWN_END -> IDLE
    IDLE -> DOWN_START [order 2] : GearshiftDown
    DOWN_BRAKE -> DOWN_END : [ticksCounter == 1]
  state Clutch_setValue(setValue) [function]
    (default) -> (junction 503)
    (junction 503) -> (junction 504) : {clutchCurrVal = setValue; send(Clutch_set);}
  note: Verifica che il controllo su min/max non sia necessario
  state EEPROM_TRIGGER [parallel]
    settings: executionOrder=6
    state WAIT
      entry:
      counterWait = 1;
      during:
      counterWait = counterWait+1;
    state SEND
      entry:
      send(eepromTrigger);
    (default) -> EEPROM_TRIGGER.WAIT
    EEPROM_TRIGGER.WAIT -> SEND : [counterWait >= 10]
    SEND -> EEPROM_TRIGGER.WAIT
  state START_ENGINE [parallel]
    settings: executionOrder=4
    state WAIT
    state START
      entry:
      send(EngineControl_start);
      lastCom = startEngCom;
      startCounter = 100;
      during:
      startCounter = startCounter - 1;
    state STOP
      entry:
      send(EngineControl_stop);
    (default) -> START_ENGINE.WAIT
    START_ENGINE.WAIT -> (junction 496)
    START_ENGINE.START -> (junction 496) [order 2] : [startEngCom != lastCom]
    (junction 496) -> START_ENGINE.START : [startEngCom != lastCom]
    STOP -> (junction 496)
    START_ENGINE.START -> STOP [order 1] : [startCounter <= 0]
  state SCAN_ADC [parallel]
    settings: executionOrder=5
    state WAIT
      entry:
      timerCounter = 0;
      during:
      timerCounter++;
    state SCAN
      entry:
      ScanADC();
    state ScanADC [function]
    (default) -> SCAN
    SCAN_ADC.WAIT -> SCAN : [timerCounter>=ADC_PERIOD]
    SCAN -> SCAN_ADC.WAIT
  state ANTISTALL_ENABLE [parallel]
    settings: executionOrder=7
    state DISABLE
      en:
      antiStallEnable = 0;
    state ENABLE
      en:
      antiStallEnable = 1;
    (default) -> DISABLE
    DISABLE -> ENABLE : [antiStall_parameters[int32(anti_stall_params.RPM_THRESHOLD)] != 0]
  note: Per ora inutile ma almeno è uno stato pronto per una futura modifica
  note: In queste transizioni vanno messi tutti i casi in cui non vogliamo parta l'antistall
  note: Verifico di aver caricato i parametri EEPROM
  data: GEAR_COMMAND_NEUTRAL_UP constant uint16 =uint16(50); GEAR_COMMAND_NEUTRAL_DOWN constant uint16 =uint16(100); GEAR_COMMAND_UP constant uint16 =uint16(400); GEAR_COMMAND_DOWN constant uint16 =uint16(200); GEAR_COMMAND_NEUTRAL_UP constant uint16 =uint16(50); GEAR_COMMAND_NEUTRAL_DOWN constant uint16 =uint16(100); GEAR_COMMAND_UP constant uint16 =uint16(400); GEAR_COMMAND_DOWN constant uint16 =uint16(200); index function_input Enum: acc_params size=1; param function_output int32 size=1; AAC_WORK_RATE_ms constant uint16 =uint16(25); aacCounter local uint16 size=1; aac_clutchValue local double size=1 =0; aac_clutchStep local double size=1; aac_dtRelease local int32 size=1; DEF_RAMP_START constant int32 =int32(50); DEF_RAMP_END constant int32 =int32(0); DEF_RAMP_TIME constant int32 =int32(250); DEF_RPM_LIMIT_1_2 constant int32 =int32(11000); DEF_RPM_LIMIT_2_3 constant int32 =int32(11000); DEF_RPM_LIMIT_3_4 constant int32 =int32(11000); DEF_RPM_LIMIT_4_5 constant int32 =int32(11000); DEF_SPEED_LIMIT_1_2 constant int32 =int32(46); DEF_SPEED_LIMIT_2_3 constant int32 =int32(61); DEF_SPEED_LIMIT_3_4 constant int32 =int32(77); DEF_SPEED_LIMIT_4_5 constant int32 =int32(113); ACC_CODE constant uint16 =uint16(1); index function_input Enum: autoX_params size=1; param function_output int32 size=1; AUTOX_WORK_RATE_ms constant uint16 =uint16(25); autoXCounter local uint16 size=1; autoX_clutchValue local double size=1 =0; autoX_clutchStep local double size=1; autoX_dtRelease local int32 size=1; lastSlip local uint16 =uint16(0); slipTarget function_input; currentSlip function_input; clutchVal function_output; reset function_input; index function_input Enum: autoX_params size=1; param function_output int32 size=1; AUTOX_WORK_RATE_ms constant uint16 =uint16(25); autoXCounter local uint16 size=1; autoX_clutchValue local double size=1 =0; autoX_clutchStep local double size=1; autoX_dtRelease local int32 size=1; lastAacCom local uint16 size=1 =uint16(0); lastShiftCom local uint16 size=1 =uint16(0); lastAutoXCom local uint16 size=1 =uint16(0); buzzerCounter local uint16 =uint8(0); time function_output int32 size=1; time function_output int32 size=1; ticksCounter local int32 size=1; data constant double; setValue function_input uint8 size=1; counterWait local double; lastCom local uint8 size=1 =uint8(0); startCounter local uint8 size=1; timerCounter local uint16; counterWait local double; currentGear input uint8 size=1 =0; clutchCurrVal output uint8 size=1 [uint8(0)..uint8(100)] =uint8(0); lastModeCom output uint16 size=2 =uint16(0); shiftCom input uint16 size=[1,2]; startEngCom input uint8 size=1; aacCom input uint16 size=[1,2]; acc_externValues input uint16 size=[1,3]; clutchTarget input uint8 size=1; lastShift local uint8 size=1 =uint8(0);; modeCom input uint16 size=[1,2]; stateFb output uint16 =uint16(0); acc_parameters input int32 size=[1,16] =aacParameters; timings input int32 size=[1,24]; autoXCom input uint16 size=[1,2]; autoX_parameters input int32 size=[1,16] =aacParameters; currSlip input uint16 size=[1,2]; antiStallEnable output uint8 size=1 =uint8(0); antiStall_parameters input int32 size=[1,8]; antiStallFb input uint16
  events: Clutch_set output FUNCTION_CALL_EVENT; Efi_init output FUNCTION_CALL_EVENT; Efi_setCut output FUNCTION_CALL_EVENT; Efi_unsetCut output FUNCTION_CALL_EVENT; Efi_setRPMLimiter output FUNCTION_CALL_EVENT; Efi_unsetRPMLimiter output FUNCTION_CALL_EVENT; Gearshift_rebound output FUNCTION_CALL_EVENT; Gearshift_up_push output FUNCTION_CALL_EVENT; Gearshift_down_push output FUNCTION_CALL_EVENT; Gearshift_brake output FUNCTION_CALL_EVENT; Gearshift_free output FUNCTION_CALL_EVENT; GearshiftUp local FUNCTION_CALL_EVENT; GearshiftDown local FUNCTION_CALL_EVENT; GearshiftSetNeutral local FUNCTION_CALL_EVENT; EngineControl_start output FUNCTION_CALL_EVENT; EngineControl_stop output FUNCTION_CALL_EVENT; eepromTrigger output FUNCTION_CALL_EVENT; BuzzerOn output FUNCTION_CALL_EVENT; BuzzerOff output FUNCTION_CALL_EVENT

== stateflow chart GCU_Model_genCode/GCU_CAN_Read/MessageEvaluation1 ==
  state sendStartEngCommand [function]
    (default) -> (junction 280)
    (junction 280) -> (junction 281) [order 1] : [startEngCommand >= 255]
    (junction 280) -> (junction 282) [order 2] : {startEngCommand = startEngCommand + 1;}
    (junction 281) -> (junction 283) : {startEngCommand = 0}
  state GEAR_RPM_TPS_UPDATE [group]
    (junction 498) -> (junction 499) : { currGear = firstInt;
        |   acc_externValues_index = uint16(acc_values.RPM);
        |   acc_externValue = secondInt;
        |   send(aac_updateExternValue);
        |   acc_externValues_index = uint16(acc_values.TPS);
        |   acc_externValue = thirdInt;
        |   send(aac_updateExternValue);}
    (junction 499) -> (junction 663) [order 1] : [RPMUpdateCounter == 255]
    (junction 499) -> (junction 667) [order 2] : {RPMUpdateCounter++;}
    (junction 663) -> (junction 665) : {RPMUpdateCounter = 0;}
  state setMap(map) [function]
  state START_ENGINE [group]
    (junction 502) -> (junction 503) : {sendStartEngCommand();}
  state sendShiftCommand(com) [function]
    note: QUESTO CONTROLLO VOGLIO SPOSTARLO IN TIMER
    (default) -> (junction 211)
    (junction 211) -> (junction 212) [order 1] : [shiftCommand[0] >= 255]
    (junction 211) -> (junction 214) [order 2] : {shiftCommand[0] = shiftCommand[0] + 1}
    (junction 212) -> (junction 215) : {shiftCommand[0] = 0}
    (junction 214) -> (junction 215)
    (junction 215) -> (junction 216) : {shiftCommand[1] = com}
    (junction 216) -> (junction 224) [order 1] : [clutchCurrVal ~= 100]
    (junction 216) -> (junction 229) [order 2]
    (junction 224) -> (junction 226)
    (junction 226) -> (junction 305) [order 1] : [(com == GEAR_COMMAND_NEUTRAL_UP) || (com == GEAR_COMMAND_NEUTRAL_DOWN) ||  (com == GEAR_COMMAND_DOWN) ]
    (junction 305) -> (junction 309) : {sendAccCommand(STOP_COM);
        |  sendAutoXCommand(AUTOX_DEFAULT);}
    (junction 226) -> (junction 307) [order 2]
  state sendStopAntiStallCommand [function] [commented out]
    (default) -> (junction 654) [commented out]
    (junction 654) -> (junction 655) [commented out] : [stopAntiStallCom >= 255]
    (junction 654) -> (junction 656) [commented out] : {stopAntiStallCom = stopAntiStallCom + 1;}
    (junction 655) -> (junction 657) [commented out] : {stopAntiStallCom = 0}
  state SW_GEARSHIFT [group]
    (junction 504) -> (junction 506) : {sendShiftCommand(firstInt);}
  state WHEEL_SPEED_UPDATE [group]
    (junction 508) -> (junction 541) : { acc_externValues_index = uint16(acc_values.WHEEL_SPEED)
        |   acc_externValue = firstInt/10;
        |   send(aac_updateExternValue);}
    (junction 541) -> (junction 670) [order 1] : [currSlip[0] >= 255]
    (junction 541) -> (junction 672) [order 2] : {currSlip++;}
    (junction 670) -> (junction 674) : {currSlip = 0;}
    (junction 672) -> (junction 674)
    (junction 674) -> (junction 677) : {currSlip = thirdInt;}
  state sendClutchCommand(com) [function] [commented out]
    (default) -> (junction 187) [commented out]
    (junction 187) -> (junction 188) [commented out] : [clutchCommand[0] >= 255]
    (junction 187) -> (junction 190) [commented out] : {clutchCommand[0] = clutchCommand[0] + 1}
    (junction 188) -> (junction 191) [commented out] : {clutchCommand[0] = 0}
    (junction 190) -> (junction 191) [commented out]
    (junction 191) -> (junction 192) [commented out] : {clutchCommand[1] = com}
  state SET_CLUTCH_MODE_MAP [group]
    (junction 511) -> (junction 512) : {clutchTarget = firstInt;
        |  sendModeCommand(secondInt);}
    (junction 512) -> (junction 552) [order 1] : [clutchTarget > CLUTCH_NOISE_LEVEL]
    (junction 512) -> (junction 553) [order 2] : {stopAntiStallCom = 0;}
    (junction 552) -> (junction 544) : {sendAccCommand(ACC_OFF);
        |  sendAutoXCommand(AUTOX_DEFAULT);
        |  stopAntiStallCom = 1; }
    (junction 553) -> (junction 544)
    (junction 544) -> (junction 548)
    (junction 548) -> (junction 632) [order 1] : [thirdInt !=0]
    (junction 548) -> (junction 636) [order 2]
    (junction 632) -> (junction 634) : {mapTarget = thirdInt;
        |  setMap(mapTarget);}
  state sendAccCommand(com) [function]
    (default) -> (junction 164)
    (junction 164) -> (junction 167) [order 1] : [accCommand[0] >= 255]
    (junction 164) -> (junction 171) [order 2] : {accCommand[0] = accCommand[0] + 1}
    (junction 167) -> (junction 173) : {accCommand[0] = 0}
    (junction 171) -> (junction 173)
    (junction 173) -> (junction 176) : {accCommand[1] = com}
  state sendAutoXCommand(com) [function]
    (default) -> (junction 598)
    (junction 598) -> (junction 599) [order 1] : [autoXCommand[0] >= 255]
    (junction 598) -> (junction 601) [order 2] : {autoXCommand[0] = autoXCommand[0] + 1}
    (junction 599) -> (junction 600) : {autoXCommand[0] = 0}
    (junction 600) -> (junction 602)
    (junction 601) -> (junction 602)
    (junction 602) -> (junction 603) : {autoXCommand[1] = com}
  state ACC_AUTOX_COM [group]
    (junction 560) -> (junction 613) [order 1] : [firstInt == ACCELERATION_MODE]
    (junction 560) -> (junction 617) [order 2]
    (junction 613) -> (junction 558) : {sendAccCommand(secondInt);}
    (junction 558) -> (junction 562) [order 1] : [accCommand[1] == ACC_OFF]
    (junction 558) -> (junction 564) [order 2]
    (junction 562) -> (junction 561) : {clutchTarget = 0;}
    (junction 617) -> (junction 627) [order 1] : [firstInt == AUTOX_MODE]
    (junction 627) -> (junction 619) : {sendAutoXCommand(secondInt);}
    (junction 617) -> (junction 629) [order 2]
    (junction 619) -> (junction 624) [order 1] : [autoXCommand[1] == AUTOX_DEFAULT]
    (junction 619) -> (junction 621) [order 2]
    (junction 624) -> (junction 620) : {clutchTarget = 0;}
  state sendModeCommand(com) [function]
    (default) -> (junction 324)
    (junction 324) -> (junction 325) [order 1] : [modeCommand[0] >= 255]
    (junction 324) -> (junction 327) [order 2] : {modeCommand[0] = modeCommand[0] + 1}
    (junction 325) -> (junction 328) : {modeCommand[0] = 0}
    (junction 327) -> (junction 328)
    (junction 328) -> (junction 329) : {modeCommand[1] = com}
  state SET_TRACTION_RPM_LIMITER [group]
    (junction 518) -> (junction 519) : {tractionTarget = uint16(firstInt);
        |  rpmLimiterTarget = uint16(secondInt);}
  note: Inserire un controllo sul minimo accettabile di map, traction, rpmLimiter
  state SET_AUTOGEARSHIFT [group]
    (junction 588) -> (junction 589)
  (default) -> (junction 389)
  (junction 389) -> (junction 498) [order 1] : [Id == EFI_GEAR_RPM_TPS_PH2O_ID]
  (junction 389) -> (junction 423) [order 2]
  (junction 423) -> (junction 502) [order 1] : [Id == SW_FIRE_GCU_ID]
  (junction 423) -> (junction 405) [order 2]
  (junction 405) -> (junction 504) [order 1] : [Id == SW_GEARSHIFT_ID]
  (junction 405) -> (junction 383) [order 2]
  (junction 383) -> (junction 508) [order 1] : [Id == EFI_TRACTION_CONTROL_ID]
  (junction 383) -> (junction 390) [order 2]
  (junction 390) -> (junction 511) [order 1] : [Id==SW_CLUTCH_MODE_MAP_GCU_ID]
  (junction 390) -> (junction 426) [order 2]
  (junction 426) -> (junction 560) [order 1] : [Id == SW_OK_BUTTON_GCU_ID]
  (junction 426) -> (junction 398) [order 2]
  (junction 398) -> (junction 518) [order 1] : [Id == SW_TRACTION_LIMITER_GCU_ID]
  (junction 398) -> (junction 586) [order 2]
  (junction 586) -> (junction 588) [order 1] : [Id==DCU_AUTOGEARSHIFT_GCU_ID]
  (junction 586) -> (junction 593) [order 2]
  data: STOP_COM constant uint16 =uint16(0); map function_input uint8; com function_input uint16 size=1; STOP_COM constant uint16 =uint16(0); GEAR_COMMAND_NEUTRAL_DOWN constant uint16 =uint16(100); GEAR_COMMAND_NEUTRAL_UP constant uint16 =uint16(50); GEAR_COMMAND_DOWN constant uint16 =uint16(200); STOP_COM constant uint16 =uint16(0); com function_input uint16 size=1; STOP_COM constant uint16 =uint16(0); CLUTCH_NOISE_LEVEL constant uint8 =uint8(30); com function_input uint16 size=1; STOP_COM constant uint16 =uint16(0); com function_input uint16 size=1; STOP_COM constant uint16 =uint16(0); com function_input uint16 size=1; Id input uint16 size=1; firstInt input uint16 size=1; secondInt input uint16 size=1; thirdInt input uint16 size=1; fourthInt input uint16 size=1; out output size=1 =0; currGear output uint16 size=1 [..uint16(5)] =uint16(0); acc_externValue output uint16 size=1 =uint16(0); acc_externValues_index output uint16 size=1 [..uint16(3)] =uint16(0); shiftCommand output uint16 size=[1, 2] =[uint16(0), uint16(0)]; startEngCommand output uint8 size=1 =uint8(0); accCommand output uint16 size=[1,2] =[uint16(0), uint16(0)]; tractionTarget output uint16 size=1; clutchTarget output uint8 size=1 =uint8(0); clutchCurrVal input uint8 size=1; modeCommand output uint16 size=[1,2] =[uint16(0), uint16(0)]; mapTarget output uint16 size=1 [..uint16(5)] =uint16(0); rpmLimiterTarget output uint16 size=1; autoXCommand output uint16 size=[1,2] =[uint16(0), uint16(0)]; stopAntiStallCom output uint8 size=1 =uint8(0); RPMUpdateCounter output uint8 size=1 =uint8(0); currSlip output uint16 size=[1,2] =[0,0]
  events: aac_updateExternValue output FUNCTION_CALL_EVENT

== stateflow chart GCU_Model_genCode/Simulink_Acc_Debug/AccelerationRoutine ==
  settings: executeAtInitialization=1
  state Wait
  state delay
    entry:
    count = 0;
    during:
    count = count + 1;
  state TPS_On
    entry:
    id = uint16(773);
    thirdInt = uint16(100);
  state ActivateAac
    entry:
    %%counter =0;
    id = uint16(514);
    firstInt = uint16(1);
    secondInt = uint16(1);
    %%during:counter = counter + 1;
  state InsertGear
    entry:
    id = uint16(512);
    firstInt = uint16(400);
    during:
    checkGear;
  state Ready
    id = uint16(514);
    firstInt = uint16(1);
    secondInt = uint16(2);
  state EnterAcceleration
    id = uint16(513);
    secondInt = uint16(1);
  state updateData [function]
    (default) -> (junction 20)
    (junction 20) -> (junction 24) [order 1] : [gearPin == 0 && lastGearPin == 1]
    (junction 20) -> (junction 22) [order 2]
    (junction 24) -> (junction 26) : { currGear = currGear + 1;}
    (junction 26) -> (junction 39)
    (junction 39) -> (junction 43)
    (junction 22) -> (junction 28) [order 1] : [gearPin == 1]
    (junction 22) -> (junction 30) [order 2] : {rpm = rpm + 150; wheelSpeed = wheelSpeed + 5;}
    (junction 28) -> (junction 33) : {rpm = 0; wheelSpeed = 0;}
    (junction 30) -> (junction 33) [order 1] : [message == 0]
    (junction 30) -> (junction 37) [order 2] : {message = 0; id = 774; firstInt = wheelSpeed;}
    (junction 33) -> (junction 35) : {message =1; id = 773; firstInt = currGear; secondInt = rpm;}
    (junction 37) -> (junction 35)
    (junction 35) -> (junction 43)
    (junction 43) -> (junction 46) : {lastGearPin = gearPin;}
  state DajeDeGas
    entry:
    id = uint16(0);
    rpm = uint16(0);
    wheelSpeed = uint16(0);
    during:
    updateData;
  state checkGear [function]
    (default) -> (junction 55)
    (junction 55) -> (junction 57) [order 1] : [gearPin == 0 && lastGearPin ==1]
    (junction 55) -> (junction 61) [order 2]
    (junction 57) -> (junction 59) : {currGear = currGear + 1;}
    (junction 59) -> (junction 64)
    (junction 61) -> (junction 64)
    (junction 64) -> (junction 67) : {lastGearPin = gearPin}
  state EXIT
    entry:
    id = uint16(513);
    firstInt = bitshift(uint16(100), 8);
  state CHANGE_MODE
    entry:
    id = uint16(1000);
    firstInt= uint16(2);
  (default) -> Wait
  Wait -> delay
  InsertGear -> TPS_On : [currGear ==1]
  delay -> EnterAcceleration : [count == 1500]
  TPS_On -> Ready
  ActivateAac -> InsertGear
  EnterAcceleration -> ActivateAac
  Ready -> DajeDeGas
  DajeDeGas -> CHANGE_MODE : [currGear == 4]
  data: id output uint16; firstInt output uint16; secondInt output uint16 =uint16(0);; counter local; gearPin input uint8; lastGearPin local uint8 =uint8(0); message local =0; rpm local uint16; wheelSpeed local uint16; currGear local uint16 =uint16(0);; count local; thirdInt output uint16 =uint16(0);
